simulink model "mpptpanel"  (R2020a)
settings: Solver=VariableStepAuto  StartTime=0.0  StopTime=10.0  FixedStep=10e-6  RelTol=1e-3
undefined symbols (not defined in the file): sigbuilder_block
libraries: powerlib x9, powerlib_meascontrol x2, re_lib x1
settings Model: Creator=ASUS  LastModifiedBy=ASUS

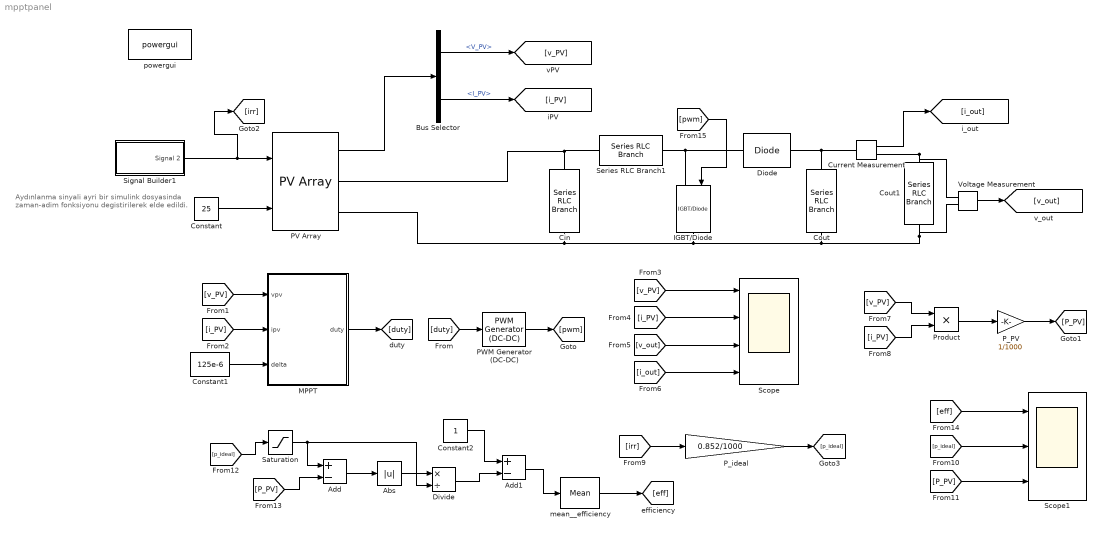
== system mpptpanel ==
  note: Aydınlanma sinyali ayri bir simulink dosyasinda
      | zaman-adim fonksiyonu degistirilerek elde edildi.
  Abs : Abs
  Add : Sum  Inputs=+-
  Add1 : Sum  Inputs=+-
  Bus Selector : BusSelector  OutputSignals=V_PV,I_PV
  Cin : powerlib/Elements/Series RLC Branch  LConnTagsString=__new0  RConnTagsString=__new0  BranchType=RC  Resistance=1e-4  Inductance=1e-3  SetiL0=off  InitialCurrent=0  Capacitance=100e-6  Setx0=off  InitialVoltage=0  Measurements=None
  Constant : Constant  Value=25
  Constant1 : Constant  Value=125e-6
  Constant2 : Constant
  Cout : powerlib/Elements/Series RLC Branch  LConnTagsString=__new0  RConnTagsString=__new0  BranchType=RC  Resistance=1e-4  Inductance=1e-3  SetiL0=off  InitialCurrent=0  Capacitance=100e-6  Setx0=off  InitialVoltage=0  Measurements=None
  Cout1 : powerlib/Elements/Series RLC Branch  LConnTagsString=__new0  RConnTagsString=__new0  BranchType=R  Resistance=20  Inductance=1e-3  SetiL0=off  InitialCurrent=0  Capacitance=100e-6  Setx0=off  InitialVoltage=0  Measurements=None
  Current Measurement : powerlib/Measurements/Current Measurement  PhasorSimulation=off  OutputType=Complex  PSBequivalent=0
  Diode : powerlib/Power Electronics/Diode  Ron=0.001  Lon=0  Vf=0.8  IC=0  UseSnubber=0  Rs=500  Cs=250e-9  Measurements=off
  Divide : Product  Inputs=*/
  IGBT/Diode : powerlib/Power Electronics/IGBT//Diode  Ron=1e-3  Rs=1e5  Cs=inf  Measurements=off
  MPPT : MATLAB Function  TreatAsAtomicUnit=on
  PV Array : re_lib/Solar/PV Array  Npar=1  Nser=1  PlotType=array @ 1000 W/m2 & specified temperatures  S_vec="[ 1000  500  100 ]"  Temp_C_vec="[ 45 25  ]"  ModuleName=SunPower SPR-X20-255  PlotWhenSelected=off  Pm=254.66  Ncell=72  Voc=51  Isc=6.3  Vm=42.8  Im=5.95  beta_Voc_pc=-0.24  alpha_Isc_pc=0.04  beta_Voc=-0.1224  alpha_Isc=0.00252  IL=6.3062  I0=1.343e-12  nI=0.94549  Rsh=449.4638  Rs=0.44063  RobustModel=off  RobustCellTemperature=25  BAL=on  Tc=1e-6  Tfilter=5e-5
  PWM Generator (DC-DC) : powerlib_meascontrol/Pulse & Signal Generators/PWM Generator (DC-DC)  Fsw=5000  Ts=5e-6
  P_PV : Gain  Gain=1/1000
  P_ideal : Gain  Gain=0.852/1000
  Product : Product
  Saturation : Saturate  UpperLimit=1000  LowerLimit=0.001
  Scope : Scope  NumInputPorts=4
  Scope1 : Scope  NumInputPorts=3
  Series RLC Branch1 : powerlib/Elements/Series RLC Branch  LConnTagsString=__new0  RConnTagsString=__new0  BranchType=RL  Resistance=0.1  Inductance=2e-3  SetiL0=off  InitialCurrent=0  Capacitance=100e-6  Setx0=off  InitialVoltage=0  Measurements=None
  Signal Builder1 : Subsystem  Tag=STV Subsys  LoadFcn=sigbuilder_block('load');  StartFcn=sigbuilder_block('start');  StopFcn=sigbuilder_block('stop');  ClipboardFcn=sigbuilder_block('clipboard');  mask(Sigbuilder block){tuvar=[0:10]}
      mask help: Simulink:masks:SigbuilderBlock_MD
      mask init:
      | if ~strcmp(get_param(bdroot(gcbh),'SimulationStatus'),'stopped') tuvar = sigbuilder_block('maskInit'); end
      settings: CopyFcn=sigbuilder_block('copy');  DeleteFcn=sigbuilder_block('delete');  ModelCloseFcn=sigbuilder_block('modelClose');  PreSaveFcn=sigbuilder_block('preSave');  PauseFcn=sigbuilder_block('pause');  ContinueFcn=sigbuilder_block('continue');  NameChangeFcn=sigbuilder_block('namechange');  OpenFcn=sigbuilder_block('open',[437.6 199.2 550.4 400 ]);  CloseFcn=sigbuilder_block('close');
      mask Display: plot(0, 0, 100, 100,[2, 2, 32, 32, 2], [68, 8, 8, 68, 68],[32, 2], [38, 38], [32, 19, 2],[53, 60, 44], [32, 17, 17, 2],[16, 16, 31, 31]);txt = getActiveGroup(gcbh);text(2, 100, txt,'verticalAlignment', 'top');
  Voltage Measurement : powerlib/Measurements/Voltage Measurement  PhasorSimulation=off  OutputType=Complex  PSBequivalent=0
  mean__efficiency : powerlib_meascontrol/Measurements/Mean  Freq=50  Vinit=0  Ts=500e-6
  powergui : powerlib/powergui  Priority=1  SimulationMode=Discrete  SampleTime=5e-6  frequency=60  Iterations=50  frequencyindice=0  Pbase=100e6  ErrMax=1e-4  UnitsV=kV  UnitsW=MW  buscounter=0  FunctionMessages=off  echomessages=off  EnableUseOfTLC=off  CurrentSourceSwitches=off  DisableSnubberDevices=off  DisableRonSwitches=off  DisableVfSwitches=off  DisplayEquations=off  AutomaticDiscreteSolvers=off  SolverType=Tustin/Backward Euler (TBE)  Interpol=off  ExternalGateDelay=off  methode=off  Ts=100  x0status=blocks  SPID=on  SwTol=0  HookPort=off  NonlinearTolerance=1e-4  nMaxIteration=100  ContinueOnMaxIteration=off  RestoreLinks=warning  ResistiveCurrentMeasurement=off  Frange=[0:2:500]  Ylog=off  Xlog=on  ShowGrid=off  save=off  variable=ZData  structure=0  ZoomFFT=off  StartTime=0.0  cycles=1  DisplayStyle=1  fundamental=60  FreqAxis=off  MaxFrequency=1000  frequencyindicesteady=1  RmsSteady=1  display=off
  wires:
  Constant/1 -> PV Array/2
  Signal Builder1/1(Signal 2) -> [irr], PV Array/1
  PV Array/1 -> Bus Selector/1
  Bus Selector/1 -> [v_PV]  "<V_PV>"
  Bus Selector/2 -> [i_PV]  "<I_PV>"
  Voltage Measurement/1 -> [v_out]
  Current Measurement/1 -> [i_out]
  [duty] -> PWM Generator (DC-DC)/1
  PWM Generator (DC-DC)/1 -> [pwm]
  Constant1/1 -> MPPT/3(delta)
  [i_PV] -> MPPT/2(ipv)
  [v_PV] -> MPPT/1(vpv)
  MPPT/1(duty) -> [duty]
  [v_PV] -> Scope/1
  [i_PV] -> Scope/2
  [v_out] -> Scope/3
  [i_out] -> Scope/4
  [v_PV] -> Product/1
  [i_PV] -> Product/2
  [irr] -> P_ideal/1
  Product/1 -> P_PV/1
  P_PV/1 -> [P_PV]
  P_ideal/1 -> [p_ideal]
  [p_ideal] -> Saturation/1
  [P_PV] -> Add/2
  Add/1 -> Abs/1
  Abs/1 -> Divide/1
  Divide/1 -> Add1/2
  Constant2/1 -> Add1/1
  Add1/1 -> mean__efficiency/1
  mean__efficiency/1 -> [eff]
  Saturation/1 -> Divide/2, Add/1
  [p_ideal] -> Scope1/2
  [P_PV] -> Scope1/3
  [eff] -> Scope1/1
  [pwm] -> IGBT/Diode/1
  connections:
  Cin/LConn1 -- Series RLC Branch1/LConn1 -- PV Array/RConn1
  Cin/RConn1 -- Voltage Measurement/LConn2 -- Cout1/RConn1 -- Cout/RConn1 -- IGBT/Diode/RConn1 -- PV Array/RConn2
  Series RLC Branch1/RConn1 -- Diode/LConn1 -- IGBT/Diode/LConn1
  Diode/RConn1 -- Current Measurement/LConn1 -- Cout/LConn1
  Current Measurement/RConn1 -- Voltage Measurement/LConn1 -- Cout1/LConn1

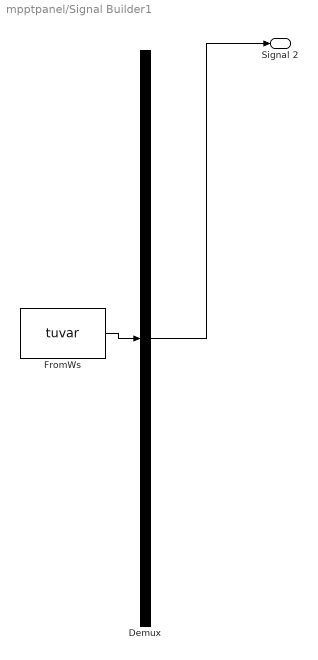
== system mpptpanel/Signal Builder1 ==
  Demux : Demux  Tag=STV Demux  Outputs=1
      settings: DisplayOption=none
  FromWs : FromWorkspace  Tag=STV FromWs  VariableName=tuvar
      SigBuilderData=|
      | common.afterFinalStr = 'Extrapolate'
      | common.sampleTime = 0
      | dataSet.timeRange = [0 30]
      | dataSet.name = 'Group 1'
      | sbobj.Groups.Name = 'Group 1'
      | sbobj.Groups.Signals.Name = 'Signal 2'
      | sbobj.Groups.Signals.XData = [0 0.0312174817898 0.0624349635796 0.0936524453694 0.124869927159 0.156087408949 0.187304890739 0.218522372529 0.249739854318 0.280957336108 0.312174817898 0.343392299688 ... (962 elements, 1x962)]
      | sbobj.Groups.Signals.YData = [2.37993 2.37993 2.37993 2.37993 2.37993 2.37993 2.37993 2.37993 2.37993 2.37992 2.37992 2.37992 ... (962 elements, 1x962)]
      | sbobj.Groups.TimeRange = [0 30]
  Signal 2 : Outport  Tag=STV Outport
  wires:
  FromWs/1 -> Demux/1
  Demux/1 -> Signal 2/1

== matlab function mpptpanel/MPPT ==
  data: vpv input; duty output; ipv input; delta input
function duty = MPPT_algorithm(vpv,ipv,delta)
duty_init = 0.1;
%duty limitlemesi gerceklestirildi
duty_min=0;
duty_max=0.85;
persistent Vold Pold duty_old;
%veri depolanmasi icin
if isempty(Vold)
    Vold=0;
    Pold=0;
    duty_old=duty_init;
end
P= vpv*ipv; %guc
dV=vpv-Vold; %gerilim degisimi
dP=P-Pold; %guc degisimi
if dP ~= 0 && vpv>30
    if dP<0
        if dV<0
            duty=duty_old - delta;
        else
            duty=duty_old + delta;
        end
    else
        if dV<0
            duty=duty_old + delta;
        else
            duty=duty_old - delta;
        end
    end
else
    duty=duty_old;
end
if duty >= duty_max
    duty=duty_max;
elseif duty<duty_min
    duty=duty_min;
end
duty_old=duty;
Vold=vpv;
Pold=P;
